simulink model "double_pendulum_simulink"  (R2020b)
settings: Solver=ode45  StartTime=0.0  StopTime=4  RelTol=1e-3
values from neighbouring files (symbols this model uses):
  g = 9.81    [double_pendulum_sim_init.m]
  l1 = 3    [double_pendulum_sim_init.m]
  l2 = 1    [double_pendulum_sim_init.m]
  m1 = 3    [double_pendulum_sim_init.m]
  m2 = 1    [double_pendulum_sim_init.m]
  teta1_i = 175*pi/180    (= 3.05432619099)    [double_pendulum_sim_init.m]
  teta1d_i = 0    [double_pendulum_sim_init.m]
  teta2_i = 180*pi/180    (= 3.14159265359)    [double_pendulum_sim_init.m]
  teta2d_i = 0    [double_pendulum_sim_init.m]
libraries: pid_lib x1
settings Model: Creator=Yigit  LastModifiedBy=Yigit

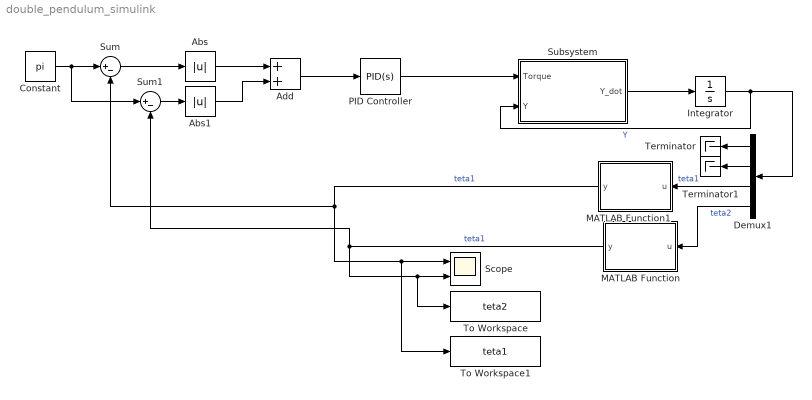
== system double_pendulum_simulink ==
  Abs : Abs
  Abs1 : Abs
  Add : Sum
  Constant : Constant  Value=pi
  Demux1 : Demux
  Integrator : Integrator  InitialCondition=[teta1d_i; teta2d_i; teta1_i; teta2_i]
  MATLAB Function : MATLAB Function  TreatAsAtomicUnit=on
  MATLAB Function1 : MATLAB Function  TreatAsAtomicUnit=on
  PID Controller : pid_lib/PID Controller  Controller=PID  Form=Parallel  TimeDomain=Continuous-time  UseExternalTs=off  SampleTime=-1  IntegratorMethod=Forward Euler  FilterMethod=Forward Euler  ControllerParametersSource=internal  P=295.994158577039  I=74.9919612861261  D=101.977488015223  UseFilter=on  N=16.0793308556286  TunerSelectOption=Transfer Function Based (PID Tuner App)  InitialConditionSource=internal  InitialConditionForIntegrator=0  InitialConditionForFilter=0  DifferentiatorICPrevScaledInput=0  ExternalReset=none  TrackingMode=off  Kt=1  LimitOutput=off  SatLimitsSource=internal  UpperSaturationLimit=inf  LowerSaturationLimit=-inf  LinearizeAsGain=on  AntiWindupMode=none  Kb=1  POutMin=[]  POutMax=[]  IOutMin=[]  IOutMax=[]  DOutMin=[]  DOutMax=[]  NOutMin=[]  NOutMax=[]  SumOutMin=[]  SumOutMax=[]  SaturationOutMin=[]  SaturationOutMax=[]  PParamMin=[]  PParamMax=[]  IParamMin=[]  IParamMax=[]  DParamMin=[]  DParamMax=[]  NParamMin=[]  NParamMax=[]  KbParamMin=[]  KbParamMax=[]  KtParamMin=[]  KtParamMax=[]  KbOutMin=[]  KbOutMax=[]  KtOutMin=[]  KtOutMax=[]  IntegratorOutMin=[]  IntegratorOutMax=[]  FilterOutMin=[]  FilterOutMax=[]  SumI1OutMin=[]  SumI1OutMax=[]  SumI2OutMin=[]  SumI2OutMax=[]  SumI3OutMin=[]  SumI3OutMax=[]  SumI4OutMin=[]  SumI4OutMax=[]  SumDOutMin=[]  SumDOutMax=[]  DifferentiatorOutMin=[]  DifferentiatorOutMax=[]  FilterDiffOutCoefMin=[]  FilterDiffOutCoefMax=[]  ReciprocalOutMin=[]  ReciprocalOutMax=[]  SumDenOutMin=[]  SumDenOutMax=[]  SumNumOutMin=[]  SumNumOutMax=[]  DivideOutMin=[]  DivideOutMax=[]  UdiffTsProdOutMin=[]  UdiffTsProdOutMax=[]  NTsProdOutMin=[]  NTsProdOutMax=[]  UintegralTsProdOutMin=[]  UintegralTsProdOutMax=[]  UngainTsProdOutMin=[]  UngainTsProdOutMax=[]  IntegratorContinuousStateAttributes=''  IntegratorStateMustResolveToSignalObject=off  IntegratorRTWStateStorageClass=Auto  FilterContinuousStateAttributes=''  FilterStateMustResolveToSignalObject=off  FilterRTWStateStorageClass=Auto  ParallelPVariant=InternalParameters  IdealPVariant=Disabled  IVariant=InternalParameters  DVariant=InternalParameters  IntegratorVariant=Continuous  SatVariant=Disabled  AWVariant=Passthrough  PCopyVariant=Disabled  TRVariant=Disabled  FdbkBlocksVariant=Forward  IdealPFdbkVariant=Disabled  SatFdbkVariant=Disabled  DerivativeFilterVariant=ContFilter  NVariant=InternalParameters  NCopyVariant=Disabled  FilterICVariant=InternalICsFilter  IntegratorICVariant=InternalICs  ExternalResetVariant=Disabled  TRSumVariant=Passthrough  SumFdbkVariant=Disabled  SumVariant=Sum_PID  TsampFilterVariant=InternalTs  TsampNgainVariant=Passthrough  TsampIntegralVariant=Passthrough  ExternalSaturationOutDataTypeStr=Inherit: Same as second input
  Scope : Scope  NumInputPorts=2
  Subsystem : Subsystem
  Sum : Sum  Inputs=|+-
  Sum1 : Sum  Inputs=|+-
  Terminator : Terminator
  Terminator1 : Terminator
  To Workspace : ToWorkspace  VariableName=teta2  SaveFormat=Timeseries  SampleTime=-1
  To Workspace1 : ToWorkspace  VariableName=teta1  SaveFormat=Timeseries  SampleTime=-1
  wires:
  Subsystem/1(Y_dot) -> Integrator/1
  PID Controller/1 -> Subsystem/1(Torque)
  Demux1/3 -> MATLAB Function1/1(u)  "teta1"
  Constant/1 -> Sum1/1, Sum/1
  Sum/1 -> Abs/1
  Abs/1 -> Add/1
  Sum1/1 -> Abs1/1
  Abs1/1 -> Add/2
  Add/1 -> PID Controller/1
  Integrator/1 -> Subsystem/2(Y), Demux1/1  "Y"
  Demux1/4 -> MATLAB Function/1(u)  "teta2"
  Demux1/2 -> Terminator1/1
  Demux1/1 -> Terminator/1
  MATLAB Function/1(y) -> To Workspace/1, Scope/2, Sum1/2  "teta1"
  MATLAB Function1/1(y) -> To Workspace1/1, Scope/1, Sum/2  "teta1"

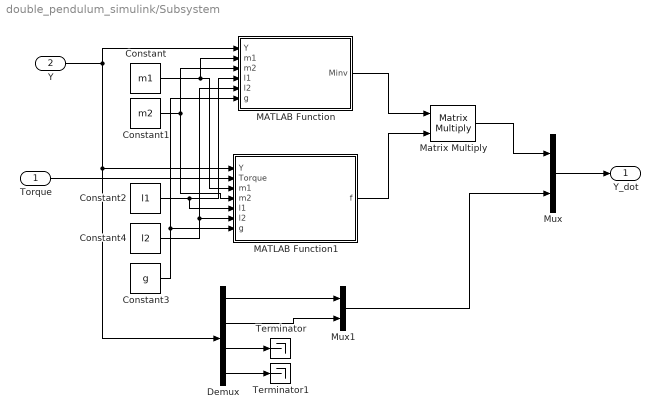
== system double_pendulum_simulink/Subsystem ==
  Torque : Inport
  Y : Inport  Port=2
  Constant : Constant  Value=m1
  Constant1 : Constant  Value=m2
  Constant2 : Constant  Value=l1
  Constant3 : Constant  Value=g
  Constant4 : Constant  Value=l2
  Demux : Demux
  MATLAB Function : MATLAB Function  TreatAsAtomicUnit=on
  MATLAB Function1 : MATLAB Function  TreatAsAtomicUnit=on
  Matrix Multiply : Product  Multiplication=Matrix(*)
  Mux : Mux  Inputs=2
  Mux1 : Mux  Inputs=2
  Terminator : Terminator
  Terminator1 : Terminator
  Y_dot : Outport
  wires:
  Demux/2 -> Mux1/2
  Matrix Multiply/1 -> Mux/1
  Demux/4 -> Terminator1/1
  Mux/1 -> Y_dot/1
  MATLAB Function/1(Minv) -> Matrix Multiply/1
  Demux/1 -> Mux1/1
  Y/1 -> Demux/1, MATLAB Function1/1(Y), MATLAB Function/1(Y)
  Mux1/1 -> Mux/2
  Demux/3 -> Terminator/1
  MATLAB Function1/1(f) -> Matrix Multiply/2
  Torque/1 -> MATLAB Function1/2(Torque)
  Constant/1 -> MATLAB Function1/3(m1), MATLAB Function/2(m1)
  Constant1/1 -> MATLAB Function1/4(m2), MATLAB Function/3(m2)
  Constant2/1 -> MATLAB Function1/5(l1), MATLAB Function/4(l1)
  Constant4/1 -> MATLAB Function1/6(l2), MATLAB Function/5(l2)
  Constant3/1 -> MATLAB Function1/7(g), MATLAB Function/6(g)

== matlab function double_pendulum_simulink/Subsystem/MATLAB Function1 ==
  data: Y input; f output; Torque input; m1 input; m2 input; l1 input; l2 input; g input
function f = Force(Y,Torque,m1,m2,l1,l2,g)
f = [ -m2*l2*Y(2)*sin(Y(3)-Y(4)) - (m1+m2)*g*sin(Y(3)) + Torque;
    l1*(Y(1)^2)*sin(Y(3)-Y(4)) - g*sin(Y(4)) ] ;

== matlab function double_pendulum_simulink/Subsystem/MATLAB Function ==
  data: Y input; Minv output; m1 input; m2 input; l1 input; l2 input; g input
function Minv = mass_matrix(Y,m1,m2,l1,l2,g)
Minv = inv([ (m1+m2)*l1 m2*l2*cos(Y(3)-Y(4));
    l1*cos(Y(3)-Y(4)) l2 ]) ;

== matlab function double_pendulum_simulink/MATLAB Function ==
  data: u input; y output
function y = fcn(u)
if u > 2*pi
    y = u - 2*pi ;
else
    y = u ;
end

== matlab function double_pendulum_simulink/MATLAB Function1 ==
  data: u input; y output
function y = fcn(u)
if u > 2*pi
    y = u - 2*pi ;
else
    y = u ;
end
